simulink model "exercicio1"  (R2015a)
settings: Solver=ode3  StartTime=0.0  StopTime=100.0  RelTol=1e-3
libraries: arduinolib x2, simulink x1
settings Model: ExtModeTrigDuration=2  Creator=Avell G1511 FIRE V3  LastModifiedBy=Avell G1511 FIRE V3
settings OptimizationCC: OptimizeModelRefInitCode=on  LifeSpan=1
settings DebuggingCC: UnderspecifiedInitializationDetection=Classic  MergeDetectMultiDrivingBlocksExec=none
settings HardwareCC: ProdBitPerInt=16  ProdBitPerPointer=8  ProdIntDivRoundTo=Zero  ProdEndianess=LittleEndian  ProdWordSize=8  ProdHWDeviceType=Atmel->AVR
settings RTWCC: SystemTargetFile=realtime.tlc  GenerateMakefile=off  TemplateMakefile=realtime.tmf  Description=Run on Target Hardware  RTWVerbose=off
settings ERTTargetCC: CombineOutputUpdateFcns=off  ExtModeTransport=3  ExtModeMexFile=ext_serial_win32_comm_rtt  ExtModeMexArgs=0 1 9600  ERTSrcFileBannerTemplate=realtime_code_template.cgt  ERTHdrFileBannerTemplate=realtime_code_template.cgt  ERTDataSrcFileTemplate=realtime_code_template.cgt  ERTDataHdrFileTemplate=realtime_code_template.cgt  ERTCustomFileTemplate=realtime_file_process.tlc

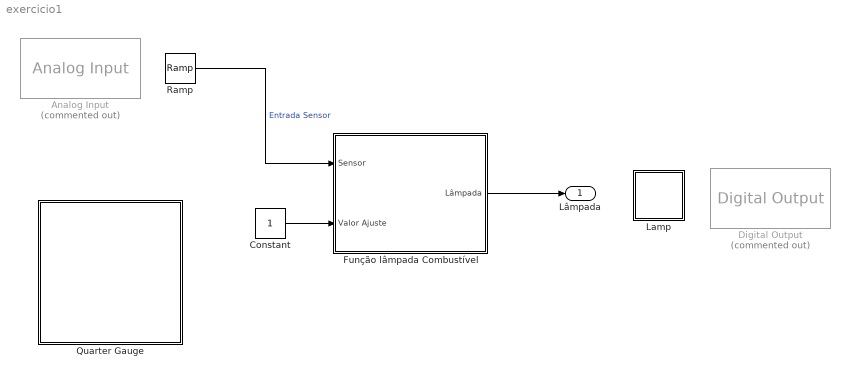
== system exercicio1 ==
  Analog Input : arduinolib/Analog Input  Commented=on  pinNumber=0  sampleTime=1  blockPlatform=arduino
  Constant : Constant
  Digital Output : arduinolib/Digital Output  Commented=on  pinNumber=9  blockPlatform=arduino
  Função lâmpada Combustível : Subsystem
  Lamp : Subsystem  DialogController=hmiCreateDDGDialog  IsWebBlock=on  mask(MathWorksWebBlock){webBlockId=6fb3120a-0d64-48c4-92eb-814f9121b9fd, webBlockType=lamp, ShowInLibBrowser=on, ShowInitialText=on, HMISrcModelName=exercicio1}
      mask prompts: webBlockType "WebBlock Type"; HMISrcModelName "Source Model"
      mask Help: helpview([docroot '/mapfiles/simulink.map'], 'hmi_lamp')
      mask Display:
      | if strcmp(get_param(bdroot(gcb),'BlockDiagramType'), 'library')
      |     image([(matlabroot) '/toolbox/simulink/hmi/icons/Lamp.png']);
      | end
  Quarter Gauge : Subsystem  DialogController=hmiCreateDDGDialog  IsWebBlock=on  mask(MathWorksWebBlock){webBlockId=7f0c22f6-f5ba-49c7-bcbb-e8fb5993d10e, webBlockType=ninetydegreegauge, ShowInLibBrowser=on, ShowInitialText=on, HMISrcModelName=exercicio1}
      mask prompts: webBlockId "WebBlock Id"; webBlockType "WebBlock Type"; HMISrcModelName "Source Model"
      mask Help: helpview([docroot '/mapfiles/simulink.map'], 'hmi_quarter_gauge')
      mask Display:
      | if strcmp(get_param(bdroot(gcb),'BlockDiagramType'), 'library')
      |     image([(matlabroot) '/toolbox/simulink/hmi/icons/NinetyDegreeGauge.png']);
      | end
  Ramp : simulink/Sources/Ramp  slope=1  start=0  X0=0
  Lâmpada : Outport
  wires:
  Ramp/1 -> Função lâmpada Combustível/1(Sensor)  "Entrada Sensor"
  Função lâmpada Combustível/1(Lâmpada) -> Lâmpada/1
  Constant/1 -> Função lâmpada Combustível/2(Valor Ajuste)

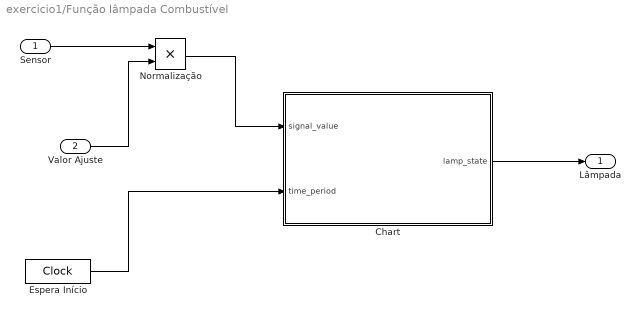
== system exercicio1/Função lâmpada Combustível ==
  Sensor : Inport
  Valor Ajuste : Inport  Port=2
  Chart : Stateflow chart  TreatAsAtomicUnit=on
  Espera Início : DigitalClock
  Normalização : Product
  Lâmpada : Outport
  wires:
  Sensor/1 -> Normalização/1
  Espera Início/1 -> Chart/2(time_period)
  Valor Ajuste/1 -> Normalização/2
  Normalização/1 -> Chart/1(signal_value)
  Chart/1(lamp_state) -> Lâmpada/1

== system exercicio1/Lamp ==

== system exercicio1/Quarter Gauge ==

== stateflow chart exercicio1/Função lâmpada Combustível/Chart ==
  state Function_Check
    entry: lamp_state = 0;
  state Lamp_On
    entry: lamp_state = 1;
  state Lamp_Off
    entry: lamp_state = 0;
  (default) -> Function_Check
  Function_Check -> Lamp_On : [time_period > 2]
  Lamp_On -> Lamp_Off : [signal_value < 8.0]
  Lamp_Off -> Lamp_On : [signal_value > 8.5]
  data: signal_value input; time_period input; lamp_state output
